simulink library "csc_peg_powered_explicit_guidance_lib"  (R2015b)
settings: Solver=VariableStepAuto  StartTime=0.0  StopTime=10.0  RelTol=1e-3
undefined symbols (not defined in the file or in its folder): accel, csc_gdn_dt, csc_peg_update_dt, DiscIntNeverNeededParam, gdn_landing_terminal_max_alt, gdn_millisec_per_cycle, gdn_peg_burn_cutoff_tgo, gdn_peg_pointing_hold_tgo, gdn_peg_Rmiss_tolerance, gdn_peg_thrust_gain, gdn_peg_Vmiss_tolerance, pos, tdl_main_biprop_thrust, tpl_main_biprop_isp, vel
libraries: util_common_lib x14, simulink x4, simulink_extras x3, util_info_lib x2, csu_arg_aimpoint_roll_guidance_lib x2, util_frame_rotation_lib x2, util_fsw_frame_rotation_lib x2, csc_peg_powered_explicit_guidance_lib x2, util_orbit_dynamics_lib x1, util_quat_lib x1
settings Model: Creator=Mark Agbayani  LastModifiedBy=Mark Agbayani

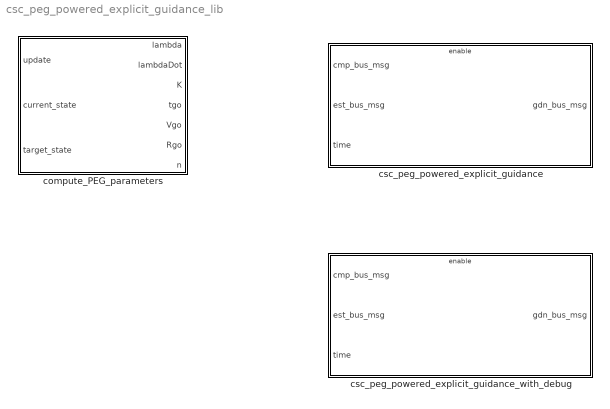
== system csc_peg_powered_explicit_guidance_lib ==
  compute_PEG_parameters : Subsystem  TreatAsAtomicUnit=on
  csc_peg_powered_explicit_guidance : Subsystem
  csc_peg_powered_explicit_guidance_with_debug : Subsystem

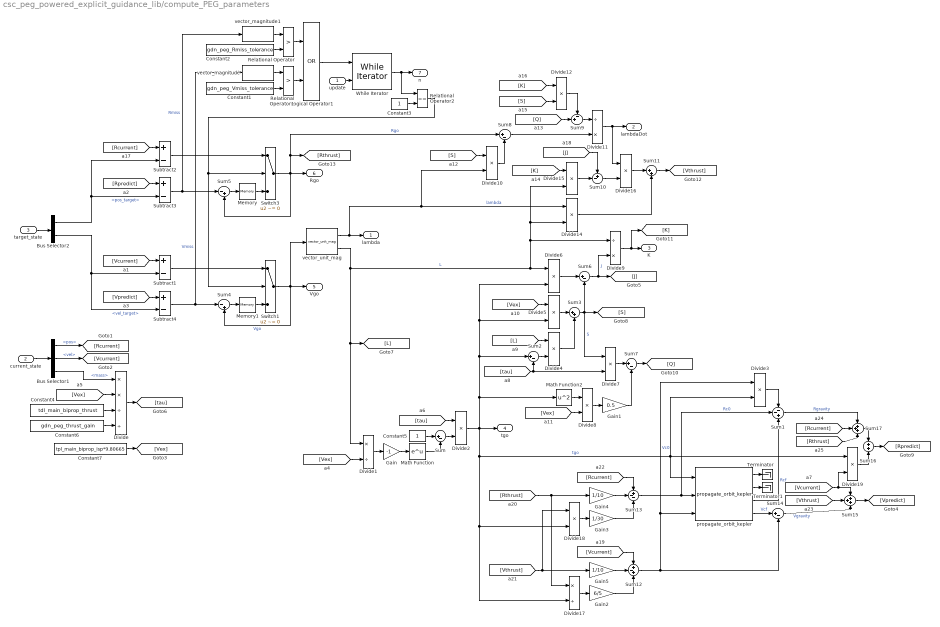
== system csc_peg_powered_explicit_guidance_lib/compute_PEG_parameters ==
  update : Inport
  current_state : Inport  Port=2
  target_state : Inport  Port=3
  Bus Selector1 : BusSelector  OutputSignals=pos,vel,mass
  Bus Selector2 : BusSelector  OutputSignals=pos_target,vel_target
  Constant1 : Constant  Value=gdn_peg_Vmiss_tolerance
  Constant2 : Constant  Value=gdn_peg_Rmiss_tolerance
  Constant3 : Constant
  Constant4 : Constant  Value=tdl_main_biprop_thrust
  Constant5 : Constant
  Constant6 : Constant  Value=gdn_peg_thrust_gain
  Constant7 : Constant  Value=tpl_main_biprop_isp*9.80665
  Divide : Product  Inputs=**//
  Divide1 : Product  Inputs=*/
  Divide{2..8,10,12,14..16,18..19} (14 alike) : Product  Inputs=**
  Divide11 : Product  Inputs=/*
  Divide17 : Product  Inputs=*/
  Divide9 : Product  Inputs=/*
  Gain : Gain  Gain=-1
  Gain1 : Gain  Gain=0.5
  Gain2 : Gain  Gain=6/5
  Gain3 : Gain  Gain=1/30
  Gain4 : Gain  Gain=1/10
  Gain5 : Gain  Gain=1/10
  Logical Operator1 : Logic  Operator=OR  AllPortsSameDT=off  OutDataTypeStr=boolean
  Math Function : Math  SaturateOnIntegerOverflow=on
  Math Function2 : Math  Operator=square  SaturateOnIntegerOverflow=on
  Memory : Memory  InheritSampleTime=on
  Memory1 : Memory  InheritSampleTime=on
  Relational Operator : RelationalOperator  Operator=>  OutDataTypeStr=boolean
  Relational Operator1 : RelationalOperator  Operator=>  OutDataTypeStr=boolean
  Relational Operator2 : RelationalOperator  Operator===  OutDataTypeStr=boolean
  Subtract{1..4} (4 alike) : Sum  Inputs=+-
  Sum{,2,6..8,14} (6 alike) : Sum  Inputs=|+-
  Sum1 : Sum  Inputs=--+
  Sum10 : Sum  Inputs=+-|
  Sum11 : Sum  Inputs=|++
  Sum12 : Sum  Inputs=+-+
  Sum13 : Sum  Inputs=+--
  Sum15 : Sum  Inputs=+++
  Sum16 : Sum  Inputs=+|+
  Sum17 : Sum  Inputs=+++
  Sum3 : Sum  Inputs=|++
  Sum4 : Sum  Inputs=|-+
  Sum5 : Sum  Inputs=|-+
  Sum9 : Sum  Inputs=-+|
  Switch1 : Switch  Criteria=u2 ~= 0
  Switch3 : Switch  Criteria=u2 ~= 0
  Terminator : Terminator
  Terminator1 : Terminator
  While Iterator : WhileIterator  MaxIters=gdn_peg_max_iterations  ResetStates=reset  ShowIterationPort=on  OutputDataType=double
  propagate_orbit_kepler : util_orbit_dynamics_lib/propagate_orbit_kepler
  vector_magnitude : util_common_lib/vector_magnitude  SystemSampleTime=-1
  vector_magnitude1 : util_common_lib/vector_magnitude  SystemSampleTime=-1
  vector_unit_mag : util_common_lib/vector_unit_mag  SystemSampleTime=-1
  lambda : Outport
  lambdaDot : Outport  Port=2
  K : Outport  Port=3
  tgo : Outport  Port=4
  Vgo : Outport  Port=5
  Rgo : Outport  Port=6
  n : Outport  Port=7
  wires:
  Constant6/1 -> Divide/4
  [Vex] -> Divide/2
  Constant4/1 -> Divide/3
  While Iterator/1 -> n/1, Relational Operator2/1
  propagate_orbit_kepler/2 -> Terminator1/1
  propagate_orbit_kepler/1 -> Terminator/1
  [Rthrust] -> Sum17/3
  [Rcurrent] -> Sum17/2
  Sum17/1 -> Sum16/1
  [Vthrust] -> Sum15/2
  Relational Operator1/1 -> Logical Operator1/2
  Relational Operator/1 -> Logical Operator1/1
  Sum15/1 -> [Vpredict]
  Sum16/1 -> [Rpredict]
  Divide19/1 -> Sum16/2
  Sum1/1 -> Sum17/1  "Rgravity"
  [Vcurrent] -> Sum15/1, Divide19/2
  Sum14/1 -> Sum15/3  "Vgravity"
  propagate_orbit_kepler/3 -> Sum1/3  "Rcf"
  Divide3/1 -> Sum1/1
  propagate_orbit_kepler/4 -> Sum14/1  "Vcf"
  Sum13/1 -> Sum1/2, propagate_orbit_kepler/2  "Rc0"
  Sum12/1 -> Sum14/2, Divide3/1, propagate_orbit_kepler/3  "Vc0"
  [Rcurrent] -> Sum13/1
  Gain3/1 -> Sum13/3
  Gain4/1 -> Sum13/2
  Gain5/1 -> Sum12/2
  Gain2/1 -> Sum12/3
  [Vcurrent] -> Sum12/1
  [Vthrust] -> Divide18/1, Gain5/1
  Divide18/1 -> Gain3/1
  [Rthrust] -> Divide17/1, Gain4/1
  Divide17/1 -> Gain2/1
  Sum11/1 -> [Vthrust]
  Divide9/1 -> K/1, [K]
  Divide15/1 -> Sum10/2
  [J] -> Sum10/1
  [K] -> Divide12/1
  [K] -> Divide15/1
  Divide14/1 -> Sum11/2
  Divide16/1 -> Sum11/1
  Sum6/1 -> [J], Divide9/2  "J"
  Sum10/1 -> Divide16/2
  Divide11/1 -> lambdaDot/1, Divide16/1
  vector_unit_mag/2 -> [L], Divide1/1, Divide6/1, Divide9/1, Divide14/2, Divide15/2  "L"
  [Q] -> Sum9/2
  Divide12/1 -> Sum9/1
  Sum9/1 -> Divide11/1
  [S] -> Divide12/2
  Sum8/1 -> Divide11/2
  Divide10/1 -> Sum8/2
  [S] -> Divide10/1
  Sum7/1 -> [Q]
  Gain1/1 -> Sum7/2
  Divide8/1 -> Gain1/1
  [Vex] -> Divide8/2
  Math Function2/1 -> Divide8/1
  Divide7/1 -> Sum7/1
  Divide6/1 -> Sum6/1
  Sum5/1 -> Memory/1
  Subtract3/1 -> Sum5/1, vector_magnitude1/1  "Rmiss"
  [Vpredict] -> Subtract4/1
  Subtract4/1 -> vector_magnitude/1, Sum4/1  "Vmiss"
  [Rpredict] -> Subtract3/1
  Sum3/1 -> Sum6/2, [S], Divide7/1  "S"
  Divide5/1 -> Sum3/1
  Divide4/1 -> Sum3/2
  [Vex] -> Divide5/1
  [L] -> Divide4/1
  Sum2/1 -> Divide4/2
  [tau] -> Divide7/2, Sum2/2
  Divide2/1 -> Math Function2/1, Sum2/1, Divide5/2, Divide6/2, propagate_orbit_kepler/1, Divide19/1, Divide3/2, Divide18/2, Divide17/2, tgo/1  "tgo"
  Math Function/1 -> Sum/2
  Constant5/1 -> Sum/1
  [tau] -> Divide2/1
  Divide1/1 -> Gain/1
  Gain/1 -> Math Function/1
  Constant7/1 -> [Vex]
  Sum/1 -> Divide2/2
  [Vex] -> Divide1/2
  Divide/1 -> [tau]
  Switch1/1 -> vector_unit_mag/1, Vgo/1, Sum4/2  "Vgo"
  Switch3/1 -> Sum5/2, Sum8/1, [Rthrust], Rgo/1  "Rgo"
  [Rcurrent] -> Subtract2/1
  [Vcurrent] -> Subtract1/1
  Bus Selector1/2 -> [Vcurrent]  "<vel>"
  Bus Selector1/1 -> [Rcurrent]  "<pos>"
  Bus Selector2/2 -> Subtract1/2, Subtract4/2  "<vel_target>"
  Bus Selector2/1 -> Subtract2/2, Subtract3/2  "<pos_target>"
  Subtract1/1 -> Switch1/1
  Subtract2/1 -> Switch3/1
  Relational Operator2/1 -> Switch1/2, Switch3/2
  Bus Selector1/3 -> Divide/1  "<mass>"
  target_state/1 -> Bus Selector2/1
  current_state/1 -> Bus Selector1/1
  Constant3/1 -> Relational Operator2/2
  vector_magnitude/1 -> Relational Operator1/1
  vector_magnitude1/1 -> Relational Operator/1
  Constant1/1 -> Relational Operator1/2
  Constant2/1 -> Relational Operator/2
  Logical Operator1/1 -> While Iterator/1
  update/1 -> While Iterator/2
  Memory/1 -> Switch3/3
  Sum4/1 -> Memory1/1
  Memory1/1 -> Switch1/3
  vector_unit_mag/1 -> lambda/1, Divide10/2, Divide14/1  "lambda"

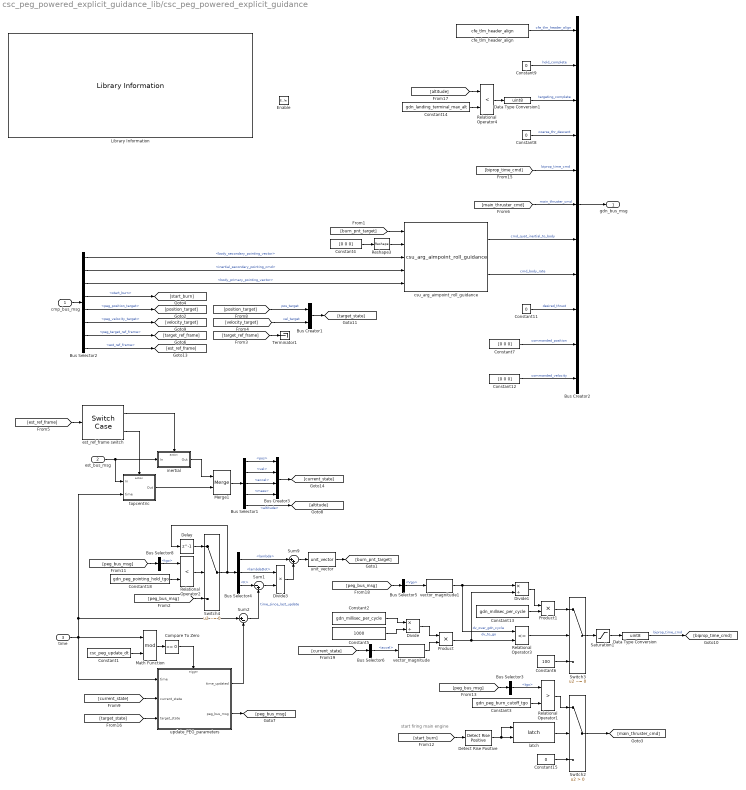
== system csc_peg_powered_explicit_guidance_lib/csc_peg_powered_explicit_guidance ==
  note: start firing main engine
  cmp_bus_msg : Inport
  est_bus_msg : Inport  Port=2
  time : Inport  Port=3
  Enable : EnablePort  StatesWhenEnabling=reset
  Bus Creator1 : BusCreator  Inputs=2
  Bus Creator3 : BusCreator  Inputs=4
  Bus Selector1 : BusSelector  OutputSignals=pos,vel,accel,mass,altitude
  Bus Selector2 : BusSelector  OutputSignals=body_secondary_pointing_vector,inertial_secondary_pointing_cmd,body_primary_pointing_vector,start_burn,peg_position_target,peg_velocity_target,peg_target_ref_frame,est_ref_frame
  Bus Selector3 : BusSelector  OutputSignals=tgo
  Bus Selector4 : BusSelector  OutputSignals=lambda,lambdaDot,K
  Bus Selector5 : BusSelector  OutputSignals=Vgo
  Bus Selector6 : BusSelector  OutputSignals=accel
  Bus Selector8 : BusSelector  OutputSignals=tgo
  Bus Creator2 : BusCreator  Inputs=11  OutDataTypeStr=Bus: gdn_bus_msg  NonVirtualBus=on
  Compare To Zero : simulink/Logic and Bit Operations/Compare To Zero  relop===  OutDataTypeStr=boolean
  Constant1 : Constant  Value=csc_peg_update_dt
  Constant11 : Constant  Value=0
  Constant12 : Constant  Value=[0 0 0]
  Constant13 : Constant  Value=gdn_millisec_per_cycle
  Constant14 : Constant  Value=gdn_landing_terminal_max_alt
  Constant15 : Constant  Value=0  OutDataTypeStr=double
  Constant18 : Constant  Value=gdn_peg_pointing_hold_tgo
  Constant2 : Constant  Value=gdn_millisec_per_cycle
  Constant3 : Constant  Value=gdn_peg_burn_cutoff_tgo
  Constant4 : Constant  Value=[0 0 0]
  Constant5 : Constant  Value=1000
  Constant6 : Constant  Value=100
  Constant7 : Constant  Value=[0 0 0]
  Constant8 : Constant  Value=0  OutDataTypeStr=uint8
  Constant9 : Constant  Value=0  OutDataTypeStr=uint8
  Data Type Conversion : DataTypeConversion  OutDataTypeStr=uint8
  Data Type Conversion1 : DataTypeConversion  OutDataTypeStr=uint8
  Delay : Delay  DelayLength=1  InitialCondition=0
  Detect Rise Positive : simulink/Logic and Bit Operations/Detect Rise Positive  vinit=0  InputProcessing=Inherited  OutDataTypeStr=boolean
  Divide : Product  Inputs=*/
  Divide1 : Product  Inputs=*/
  Divide3 : Product  Inputs=**  OutDataTypeStr=double
  Library Information : util_info_lib/Library Information  owner='jkaidy'
  Math Function : Math  Operator=mod  SaturateOnIntegerOverflow=on
  Merge1 : Merge  InitialOutput=0
  Product : Product
  Product1 : Product
  Relational Operator1 : RelationalOperator  Operator=>  OutDataTypeStr=boolean
  Relational Operator2 : RelationalOperator  Operator=<  OutDataTypeStr=boolean
  Relational Operator3 : RelationalOperator  Operator=<=  OutDataTypeStr=boolean
  Relational Operator4 : RelationalOperator  Operator=<  OutDataTypeStr=boolean
  Reshape3 : Reshape  OutputDimensionality=Column vector (2-D)
  Saturation1 : Saturate  UpperLimit=100  LowerLimit=0
  Sum1 : Sum  Inputs=|-+  AccumDataTypeStr=double
  Sum2 : Sum  Inputs=|+-
  Sum9 : Sum  Inputs=|++  AccumDataTypeStr=double
  Switch2 : Switch  Criteria=u2 > Threshold
  Switch3 : Switch  Criteria=u2 ~= 0
  Switch4 : Switch  Criteria=u2 ~= 0  OutDataTypeStr=double
  Terminator1 : Terminator
  cfe_tlm_header_align : util_common_lib/cfe_tlm_header_align
  csu_arg_aimpoint_roll_guidance : csu_arg_aimpoint_roll_guidance_lib/csu_arg_aimpoint_roll_guidance
  est_ref_frame switch : SwitchCase  CaseConditions={uint8(enum_reference_frame.inertial),uint8(enum_reference_frame.topocentric)}  ShowDefaultCase=off
  inertial : Subsystem  TreatAsAtomicUnit=on
  latch : util_common_lib/latch  Initial_Latch=0
  topcentric : Subsystem  TreatAsAtomicUnit=on
  unit_vector : util_common_lib/unit_vector  SystemSampleTime=-1
  update_PEG_parameters : Subsystem  TreatAsAtomicUnit=on
  vector_magnitude : util_common_lib/vector_magnitude  SystemSampleTime=-1
  vector_magnitude1 : util_common_lib/vector_magnitude  SystemSampleTime=-1
  gdn_bus_msg : Outport  OutDataTypeStr=Bus: gdn_bus_msg
  wires:
  Merge1/1 -> Bus Selector1/1
  [est_ref_frame] -> est_ref_frame switch/1
  time/1 -> update_PEG_parameters/1(time), Math Function/1, Sum2/1, topcentric/2(time)
  est_ref_frame switch/2 -> topcentric/Action
  topcentric/1(Out) -> Merge1/2
  inertial/1(Out) -> Merge1/1
  est_bus_msg/1 -> inertial/1(In), topcentric/1(In)
  est_ref_frame switch/1 -> inertial/Action
  [current_state] -> Bus Selector6/1
  Bus Creator3/1 -> [current_state]
  Bus Selector1/1 -> Bus Creator3/1  "<pos>"
  Bus Selector1/2 -> Bus Creator3/2  "<vel>"
  Bus Selector1/3 -> Bus Creator3/3  "<accel>"
  Bus Selector2/8 -> [est_ref_frame]  "<est_ref_frame>"
  Bus Selector2/7 -> [target_ref_frame]  "<peg_target_ref_frame>"
  Bus Creator1/1 -> [target_state]
  [position_target] -> Bus Creator1/1  "pos_target"
  [velocity_target] -> Bus Creator1/2  "vel_target"
  [target_ref_frame] -> Terminator1/1
  [biprop_time_cmd] -> Bus Creator2/5  "biprop_time_cmd"
  cmp_bus_msg/1 -> Bus Selector2/1
  Bus Selector2/5 -> [position_target]  "<peg_position_target>"
  Bus Selector2/6 -> [velocity_target]  "<peg_velocity_target>"
  Bus Selector2/1 -> csu_arg_aimpoint_roll_guidance/3  "<body_secondary_pointing_vector>"
  Bus Selector2/2 -> csu_arg_aimpoint_roll_guidance/4  "<inertial_secondary_pointing_cmd>"
  Bus Selector2/3 -> csu_arg_aimpoint_roll_guidance/5  "<body_primary_pointing_vector>"
  Bus Selector2/4 -> [start_burn]  "<start_burn>"
  Constant11/1 -> Bus Creator2/9  "desired_thrust"
  Constant8/1 -> Bus Creator2/4  "coarse_thr_descent"
  [main_thruster_cmd] -> Bus Creator2/6  "main_thruster_cmd"
  csu_arg_aimpoint_roll_guidance/1 -> Bus Creator2/7  "cmd_quat_inertial_to_body"
  csu_arg_aimpoint_roll_guidance/2 -> Bus Creator2/8  "cmd_body_rate"
  Constant9/1 -> Bus Creator2/2  "hold_complete"
  Data Type Conversion1/1 -> Bus Creator2/3  "targeting_complete"
  cfe_tlm_header_align/1 -> Bus Creator2/1  "cfe_tlm_header_align"
  Constant12/1 -> Bus Creator2/11  "commanded_velocity"
  Constant7/1 -> Bus Creator2/10  "commanded_position"
  Detect Rise Positive/1 -> latch/1, latch/2
  [start_burn] -> Detect Rise Positive/1
  Constant3/1 -> Relational Operator1/2
  Relational Operator1/1 -> Switch2/1
  Constant15/1 -> Switch2/3
  Switch2/1 -> [main_thruster_cmd]
  latch/1 -> Switch2/2
  Bus Selector1/4 -> Bus Creator3/4  "<mass>"
  [burn_pnt_target] -> csu_arg_aimpoint_roll_guidance/1
  Reshape3/1 -> csu_arg_aimpoint_roll_guidance/2
  Constant4/1 -> Reshape3/1
  [current_state] -> update_PEG_parameters/2(current_state)
  [target_state] -> update_PEG_parameters/3(target_state)
  Bus Selector3/1 -> Relational Operator1/1  "<tgo>"
  [peg_bus_msg] -> Bus Selector3/1
  update_PEG_parameters/2(peg_bus_msg) -> [peg_bus_msg]
  Math Function/1 -> Compare To Zero/1
  Constant1/1 -> Math Function/2
  update_PEG_parameters/1(time_updated) -> Sum2/2
  Data Type Conversion/1 -> [biprop_time_cmd]  "biprop_time_cmd"
  Saturation1/1 -> Data Type Conversion/1
  vector_magnitude/1 -> Product/2
  Switch3/1 -> Saturation1/1
  Product1/1 -> Switch3/1
  Divide1/1 -> Product1/1
  Constant13/1 -> Product1/2
  Product/1 -> Relational Operator3/2, Divide1/2  "dv_over_gdn_cycle"
  Constant6/1 -> Switch3/3
  Relational Operator3/1 -> Switch3/2
  vector_magnitude1/1 -> Relational Operator3/1, Divide1/1  "dv_to_go"
  Bus Selector6/1 -> vector_magnitude/1  "<accel>"
  Divide/1 -> Product/1
  Constant5/1 -> Divide/2
  Constant2/1 -> Divide/1
  [peg_bus_msg] -> Bus Selector5/1
  Bus Selector5/1 -> vector_magnitude1/1  "<Vgo>"
  Bus Creator2/1 -> gdn_bus_msg/1
  Compare To Zero/1 -> update_PEG_parameters/Trigger
  unit_vector/1 -> [burn_pnt_target]
  Bus Selector1/5 -> [altitude]  "<altitude>"
  [altitude] -> Relational Operator4/1
  Constant14/1 -> Relational Operator4/2
  Relational Operator4/1 -> Data Type Conversion1/1
  Sum2/1 -> Sum1/2  "time_since_last_update"
  Switch4/1 -> Delay/1, Bus Selector4/1
  Sum1/1 -> Divide3/2
  Divide3/1 -> Sum9/2
  Bus Selector4/3 -> Sum1/1  "<K>"
  Bus Selector4/2 -> Divide3/1  "<lambdaDot>"
  Bus Selector4/1 -> Sum9/1  "<lambda>"
  Sum9/1 -> unit_vector/1
  Bus Selector8/1 -> Relational Operator2/1  "<tgo>"
  [peg_bus_msg] -> Bus Selector8/1
  Constant18/1 -> Relational Operator2/2
  Delay/1 -> Switch4/1
  Relational Operator2/1 -> Switch4/2
  [peg_bus_msg] -> Switch4/3

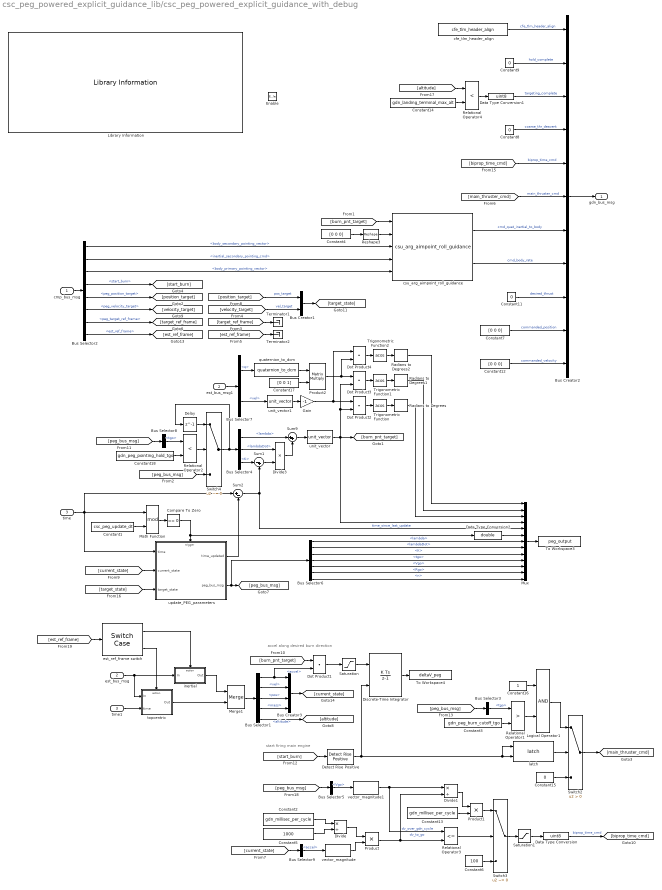
== system csc_peg_powered_explicit_guidance_lib/csc_peg_powered_explicit_guidance_with_debug ==
  note: accel along desired burn direction
  note: start firing main engine
  cmp_bus_msg : Inport
  est_bus_msg : Inport  Port=2
  time : Inport  Port=3
  Enable : EnablePort  StatesWhenEnabling=reset
  Bus Creator1 : BusCreator  Inputs=2
  Bus Creator3 : BusCreator  Inputs=4
  Bus Selector1 : BusSelector  OutputSignals=accel,vel,pos,mass,altitude
  Bus Selector2 : BusSelector  OutputSignals=body_secondary_pointing_vector,inertial_secondary_pointing_cmd,body_primary_pointing_vector,start_burn,peg_position_target,peg_velocity_target,peg_target_ref_frame,est_ref_frame
  Bus Selector3 : BusSelector  OutputSignals=tgo
  Bus Selector4 : BusSelector  OutputSignals=lambda,lambdaDot,K
  Bus Selector5 : BusSelector  OutputSignals=Vgo
  Bus Selector6 : BusSelector  OutputSignals=lambda,lambdaDot,K,tgo,Vgo,Rgo,n
  Bus Selector7 : BusSelector  OutputSignals=q,vel
  Bus Selector8 : BusSelector  OutputSignals=tgo
  Bus Selector9 : BusSelector  OutputSignals=accel
  Bus Creator2 : BusCreator  Inputs=11  OutDataTypeStr=Bus: gdn_bus_msg  NonVirtualBus=on
  Compare To Zero : simulink/Logic and Bit Operations/Compare To Zero  relop===  OutDataTypeStr=boolean
  Constant1 : Constant  Value=csc_peg_update_dt
  Constant11 : Constant  Value=0
  Constant12 : Constant  Value=[0 0 0]
  Constant13 : Constant  Value=gdn_millisec_per_cycle
  Constant14 : Constant  Value=gdn_landing_terminal_max_alt
  Constant15 : Constant  Value=0  OutDataTypeStr=double
  Constant16 : Constant  OutDataTypeStr=boolean
  Constant17 : Constant  Value=[0 0 1]
  Constant18 : Constant  Value=gdn_peg_pointing_hold_tgo
  Constant2 : Constant  Value=gdn_millisec_per_cycle
  Constant3 : Constant  Value=gdn_peg_burn_cutoff_tgo
  Constant4 : Constant  Value=[0 0 0]
  Constant5 : Constant  Value=1000
  Constant6 : Constant  Value=100
  Constant7 : Constant  Value=[0 0 0]
  Constant8 : Constant  Value=0  OutDataTypeStr=uint8
  Constant9 : Constant  Value=0  OutDataTypeStr=uint8
  Data Type Conversion : DataTypeConversion  OutDataTypeStr=uint8
  Data Type Conversion1 : DataTypeConversion  OutDataTypeStr=uint8
  Data Type Conversion2 : DataTypeConversion  OutDataTypeStr=double
  Delay : Delay  DelayLength=1  InitialCondition=0
  Detect Rise Positive : simulink/Logic and Bit Operations/Detect Rise Positive  vinit=0  InputProcessing=Inherited  OutDataTypeStr=boolean
  Discrete-Time Integrator : DiscreteIntegrator  ExternalReset=rising  SampleTime=csc_gdn_dt  ICPrevOutput=DiscIntNeverNeededParam  ICPrevScaledInput=DiscIntNeverNeededParam
  Divide : Product  Inputs=*/
  Divide1 : Product  Inputs=*/
  Divide3 : Product  Inputs=**  OutDataTypeStr=double
  Dot Product{1..4} (4 alike) : DotProduct  InputSameDT=on  OutDataTypeStr=Inherit: Inherit via internal rule
  Gain : Gain  Gain=-1
  Library Information : util_info_lib/Library Information  owner='jkaidy'
  Logical Operator1 : Logic  AllPortsSameDT=off  OutDataTypeStr=boolean
  Math Function : Math  Operator=mod  SaturateOnIntegerOverflow=on
  Merge1 : Merge  InitialOutput=0
  Mux : Mux  Inputs=13
  Product : Product
  Product1 : Product
  Product2 : Product  Multiplication=Matrix(*)  RndMeth=Zero
  Radians to Degrees : simulink_extras/Transformations/Radians to Degrees
  Radians to Degrees1 : simulink_extras/Transformations/Radians to Degrees
  Radians to Degrees2 : simulink_extras/Transformations/Radians to Degrees
  Relational Operator1 : RelationalOperator  Operator=>  OutDataTypeStr=boolean
  Relational Operator2 : RelationalOperator  Operator=<  OutDataTypeStr=boolean
  Relational Operator3 : RelationalOperator  Operator=<=  OutDataTypeStr=boolean
  Relational Operator4 : RelationalOperator  Operator=<  OutDataTypeStr=boolean
  Reshape3 : Reshape  OutputDimensionality=Column vector (2-D)
  Saturation : Saturate  UpperLimit=1e6  LowerLimit=0
  Saturation1 : Saturate  UpperLimit=100  LowerLimit=0
  Sum1 : Sum  Inputs=|-+  AccumDataTypeStr=double
  Sum2 : Sum  Inputs=|+-
  Sum9 : Sum  Inputs=|++  AccumDataTypeStr=double
  Switch2 : Switch  Criteria=u2 > Threshold
  Switch3 : Switch  Criteria=u2 ~= 0
  Switch4 : Switch  Criteria=u2 ~= 0  OutDataTypeStr=double
  Terminator1 : Terminator
  Terminator2 : Terminator
  To Workspace3 : ToWorkspace  VariableName=peg_output  SaveFormat=Structure With Time  SampleTime=-1
  To Workspace4 : ToWorkspace  VariableName=deltaV_peg  SaveFormat=Structure With Time  SampleTime=-1
  Trigonometric Function : Trigonometry  Operator=acos
  Trigonometric Function1 : Trigonometry  Operator=acos
  Trigonometric Function2 : Trigonometry  Operator=acos
  cfe_tlm_header_align : util_common_lib/cfe_tlm_header_align
  csu_arg_aimpoint_roll_guidance : csu_arg_aimpoint_roll_guidance_lib/csu_arg_aimpoint_roll_guidance
  est_bus_msg1 : InportShadow  Port=2
  est_ref_frame switch : SwitchCase  CaseConditions={uint8(enum_reference_frame.inertial),uint8(enum_reference_frame.topocentric)}  ShowDefaultCase=off
  inertial : Subsystem  TreatAsAtomicUnit=on
  latch : util_common_lib/latch  Initial_Latch=0
  quaternion_to_dcm : util_quat_lib/quaternion_to_dcm  SystemSampleTime=-1
  time1 : InportShadow  Port=3
  topcentric : Subsystem  TreatAsAtomicUnit=on
  unit_vector : util_common_lib/unit_vector  SystemSampleTime=-1
  unit_vector1 : util_common_lib/unit_vector  SystemSampleTime=-1
  update_PEG_parameters : Subsystem  TreatAsAtomicUnit=on
  vector_magnitude : util_common_lib/vector_magnitude  SystemSampleTime=-1
  vector_magnitude1 : util_common_lib/vector_magnitude  SystemSampleTime=-1
  gdn_bus_msg : Outport  OutDataTypeStr=Bus: gdn_bus_msg
  wires:
  [current_state] -> Bus Selector9/1
  time1/1 -> topcentric/2(time)
  Bus Selector1/1 -> Bus Creator3/1, Dot Product1/2  "<accel>"
  Bus Selector1/2 -> Bus Creator3/2  "<vel>"
  Bus Selector1/3 -> Bus Creator3/3  "<pos>"
  [est_ref_frame] -> Terminator2/1
  Bus Selector2/8 -> [est_ref_frame]  "<est_ref_frame>"
  Constant16/1 -> Logical Operator1/1
  Relational Operator1/1 -> Logical Operator1/2
  [peg_bus_msg] -> Bus Selector3/1
  Bus Selector3/1 -> Relational Operator1/1  "<tgo>"
  Constant3/1 -> Relational Operator1/2
  Dot Product4/1 -> Trigonometric Function2/1
  Trigonometric Function2/1 -> Radians to Degrees2/1
  Saturation/1 -> Discrete-Time Integrator/1
  [burn_pnt_target] -> Dot Product1/1
  Dot Product1/1 -> Saturation/1
  Detect Rise Positive/1 -> latch/2, latch/1, Discrete-Time Integrator/2
  Discrete-Time Integrator/1 -> To Workspace4/1
  update_PEG_parameters/2(peg_bus_msg) -> [peg_bus_msg], Bus Selector6/1
  Sum2/1 -> Sum1/2, Mux/5  "time_since_last_update"
  Mux/1 -> To Workspace3/1
  unit_vector/1 -> Dot Product3/2, Dot Product2/2, [burn_pnt_target], Mux/4
  Bus Selector6/1 -> Mux/7  "<lambda>"
  Bus Selector6/2 -> Mux/8  "<lambdaDot>"
  Bus Selector6/3 -> Mux/9  "<K>"
  Bus Selector6/4 -> Mux/10  "<tgo>"
  Bus Selector6/5 -> Mux/11  "<Vgo>"
  Bus Selector6/6 -> Mux/12  "<Rgo>"
  Bus Selector6/7 -> Mux/13  "<n>"
  Compare To Zero/1 -> update_PEG_parameters/Trigger, Data Type Conversion2/1
  Data Type Conversion2/1 -> Mux/6
  est_bus_msg1/1 -> Bus Selector7/1
  Bus Selector7/2 -> unit_vector1/1  "<vel>"
  unit_vector1/1 -> Gain/1
  Dot Product2/1 -> Trigonometric Function/1
  Trigonometric Function/1 -> Radians to Degrees/1
  Radians to Degrees/1 -> Mux/3
  Gain/1 -> Dot Product2/1, Dot Product4/1
  Bus Selector7/1 -> quaternion_to_dcm/1  "<q>"
  quaternion_to_dcm/1 -> Product2/1
  Constant17/1 -> Product2/2
  Dot Product3/1 -> Trigonometric Function1/1
  Trigonometric Function1/1 -> Radians to Degrees1/1
  Radians to Degrees1/1 -> Mux/2
  Product2/1 -> Dot Product4/2, Dot Product3/1
  Radians to Degrees2/1 -> Mux/1
  [target_ref_frame] -> Terminator1/1
  Bus Selector2/6 -> [velocity_target]  "<peg_velocity_target>"
  Bus Selector2/7 -> [target_ref_frame]  "<peg_target_ref_frame>"
  Bus Selector2/5 -> [position_target]  "<peg_position_target>"
  Bus Creator2/1 -> gdn_bus_msg/1
  Bus Selector5/1 -> vector_magnitude1/1  "<Vgo>"
  [peg_bus_msg] -> Bus Selector5/1
  Constant2/1 -> Divide/1
  Constant5/1 -> Divide/2
  Divide/1 -> Product/1
  Bus Selector9/1 -> vector_magnitude/1  "<accel>"
  Product/1 -> Relational Operator3/2, Divide1/2  "dv_over_gdn_cycle"
  vector_magnitude1/1 -> Divide1/1, Relational Operator3/1  "dv_to_go"
  Relational Operator3/1 -> Switch3/2
  Constant6/1 -> Switch3/3
  Constant13/1 -> Product1/2
  Divide1/1 -> Product1/1
  Product1/1 -> Switch3/1
  Switch3/1 -> Saturation1/1
  vector_magnitude/1 -> Product/2
  Saturation1/1 -> Data Type Conversion/1
  Data Type Conversion/1 -> [biprop_time_cmd]  "biprop_time_cmd"
  update_PEG_parameters/1(time_updated) -> Sum2/2
  time/1 -> Sum2/1, Math Function/1, update_PEG_parameters/1(time)
  Constant1/1 -> Math Function/2
  Math Function/1 -> Compare To Zero/1
  [velocity_target] -> Bus Creator1/2  "vel_target"
  [position_target] -> Bus Creator1/1  "pos_target"
  Bus Creator1/1 -> [target_state]
  [target_state] -> update_PEG_parameters/3(target_state)
  [current_state] -> update_PEG_parameters/2(current_state)
  Constant4/1 -> Reshape3/1
  Reshape3/1 -> csu_arg_aimpoint_roll_guidance/2
  [burn_pnt_target] -> csu_arg_aimpoint_roll_guidance/1
  latch/1 -> Switch2/2
  Switch2/1 -> [main_thruster_cmd]
  Constant15/1 -> Switch2/3
  Logical Operator1/1 -> Switch2/1
  [start_burn] -> Detect Rise Positive/1
  Constant7/1 -> Bus Creator2/10  "commanded_position"
  Constant12/1 -> Bus Creator2/11  "commanded_velocity"
  cfe_tlm_header_align/1 -> Bus Creator2/1  "cfe_tlm_header_align"
  Data Type Conversion1/1 -> Bus Creator2/3  "targeting_complete"
  csu_arg_aimpoint_roll_guidance/2 -> Bus Creator2/8  "cmd_body_rate"
  csu_arg_aimpoint_roll_guidance/1 -> Bus Creator2/7  "cmd_quat_inertial_to_body"
  [main_thruster_cmd] -> Bus Creator2/6  "main_thruster_cmd"
  Constant8/1 -> Bus Creator2/4  "coarse_thr_descent"
  Constant11/1 -> Bus Creator2/9  "desired_thrust"
  Bus Selector2/4 -> [start_burn]  "<start_burn>"
  Bus Selector2/3 -> csu_arg_aimpoint_roll_guidance/5  "<body_primary_pointing_vector>"
  Bus Selector2/2 -> csu_arg_aimpoint_roll_guidance/4  "<inertial_secondary_pointing_cmd>"
  Bus Selector2/1 -> csu_arg_aimpoint_roll_guidance/3  "<body_secondary_pointing_vector>"
  cmp_bus_msg/1 -> Bus Selector2/1
  [biprop_time_cmd] -> Bus Creator2/5  "biprop_time_cmd"
  [altitude] -> Relational Operator4/1
  Constant14/1 -> Relational Operator4/2
  Relational Operator4/1 -> Data Type Conversion1/1
  Constant9/1 -> Bus Creator2/2  "hold_complete"
  Switch4/1 -> Delay/1, Bus Selector4/1
  Sum1/1 -> Divide3/2
  Divide3/1 -> Sum9/2
  Bus Selector4/3 -> Sum1/1  "<K>"
  Bus Selector4/2 -> Divide3/1  "<lambdaDot>"
  Bus Selector4/1 -> Sum9/1  "<lambda>"
  Sum9/1 -> unit_vector/1
  Bus Selector8/1 -> Relational Operator2/1  "<tgo>"
  [peg_bus_msg] -> Bus Selector8/1
  Constant18/1 -> Relational Operator2/2
  Delay/1 -> Switch4/1
  Relational Operator2/1 -> Switch4/2
  [peg_bus_msg] -> Switch4/3
  Bus Selector1/5 -> [altitude]  "<altitude>"
  Bus Selector1/4 -> Bus Creator3/4  "<mass>"
  Bus Creator3/1 -> [current_state]
  est_ref_frame switch/1 -> inertial/Action
  est_bus_msg/1 -> topcentric/1(In), inertial/1(In)
  inertial/1(Out) -> Merge1/1
  topcentric/1(Out) -> Merge1/2
  est_ref_frame switch/2 -> topcentric/Action
  [est_ref_frame] -> est_ref_frame switch/1
  Merge1/1 -> Bus Selector1/1

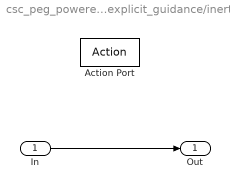
== system csc_peg_powered_explicit_guidance_lib/csc_peg_powered_explicit_guidance/inertial ==
  In : Inport
  Action Port : ActionPort
  Out : Outport
  wires:
  In/1 -> Out/1

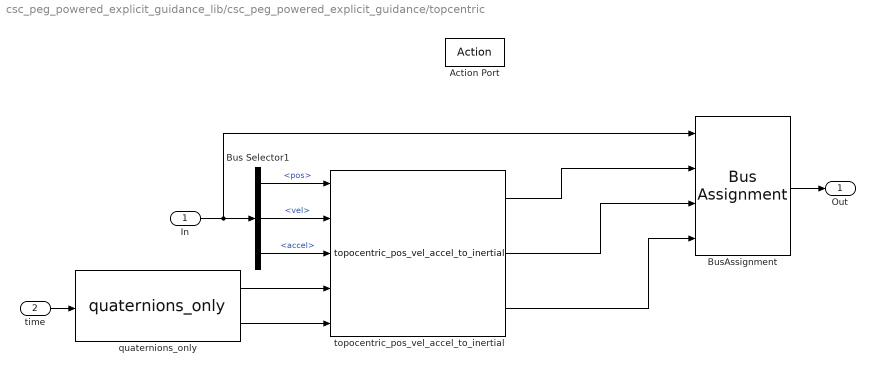
== system csc_peg_powered_explicit_guidance_lib/csc_peg_powered_explicit_guidance/topcentric ==
  In : Inport
  time : Inport  Port=2
  Action Port : ActionPort
  Bus Selector1 : BusSelector  OutputSignals=pos,vel,accel
  BusAssignment : BusAssignment  AssignedSignals=pos,vel,accel
  quaternions_only : util_frame_rotation_lib/quaternions_only  SystemSampleTime=-1
  topocentric_pos_vel_accel_to_inertial : util_fsw_frame_rotation_lib/topocentric_pos_vel_accel_to_inertial  SystemSampleTime=-1
  Out : Outport
  wires:
  quaternions_only/2 -> topocentric_pos_vel_accel_to_inertial/5
  quaternions_only/1 -> topocentric_pos_vel_accel_to_inertial/4
  time/1 -> quaternions_only/1
  BusAssignment/1 -> Out/1
  topocentric_pos_vel_accel_to_inertial/3 -> BusAssignment/4
  topocentric_pos_vel_accel_to_inertial/2 -> BusAssignment/3
  topocentric_pos_vel_accel_to_inertial/1 -> BusAssignment/2
  In/1 -> Bus Selector1/1, BusAssignment/1
  Bus Selector1/3 -> topocentric_pos_vel_accel_to_inertial/3  "<accel>"
  Bus Selector1/2 -> topocentric_pos_vel_accel_to_inertial/2  "<vel>"
  Bus Selector1/1 -> topocentric_pos_vel_accel_to_inertial/1  "<pos>"

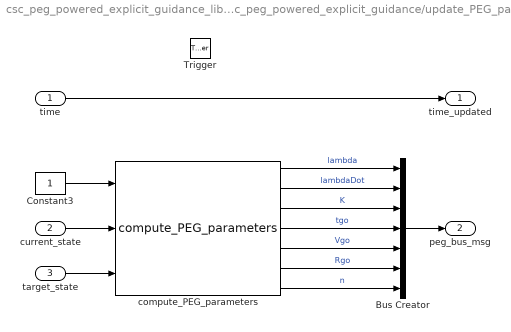
== system csc_peg_powered_explicit_guidance_lib/csc_peg_powered_explicit_guidance/update_PEG_parameters ==
  time : Inport
  current_state : Inport  Port=2
  target_state : Inport  Port=3
  Trigger : TriggerPort  TriggerType=falling
  Bus Creator : BusCreator  Inputs=7
  Constant3 : Constant
  compute_PEG_parameters : csc_peg_powered_explicit_guidance_lib/compute_PEG_parameters
  time_updated : Outport
  peg_bus_msg : Outport  Port=2
  wires:
  compute_PEG_parameters/4 -> Bus Creator/4  "tgo"
  compute_PEG_parameters/7 -> Bus Creator/7  "n"
  compute_PEG_parameters/6 -> Bus Creator/6  "Rgo"
  compute_PEG_parameters/5 -> Bus Creator/5  "Vgo"
  compute_PEG_parameters/3 -> Bus Creator/3  "K"
  compute_PEG_parameters/2 -> Bus Creator/2  "lambdaDot"
  compute_PEG_parameters/1 -> Bus Creator/1  "lambda"
  Bus Creator/1 -> peg_bus_msg/1
  current_state/1 -> compute_PEG_parameters/2
  target_state/1 -> compute_PEG_parameters/3
  Constant3/1 -> compute_PEG_parameters/1
  time/1 -> time_updated/1

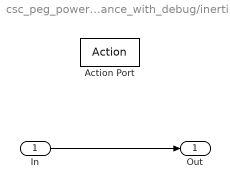
== system csc_peg_powered_explicit_guidance_lib/csc_peg_powered_explicit_guidance_with_debug/inertial ==
  In : Inport
  Action Port : ActionPort
  Out : Outport
  wires:
  In/1 -> Out/1

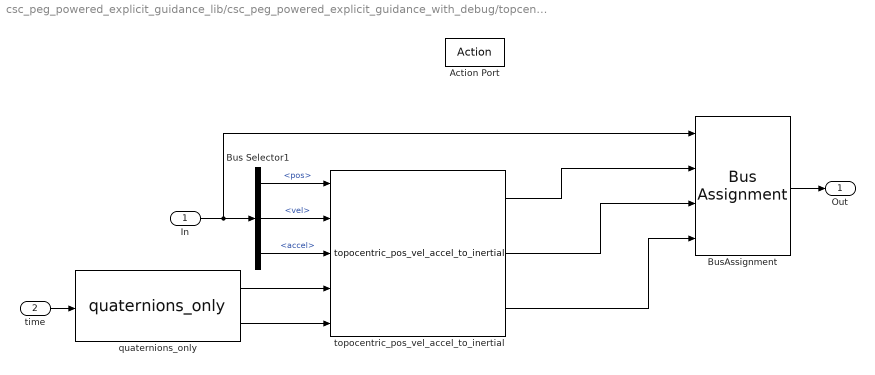
== system csc_peg_powered_explicit_guidance_lib/csc_peg_powered_explicit_guidance_with_debug/topcentric ==
  In : Inport
  time : Inport  Port=2
  Action Port : ActionPort
  Bus Selector1 : BusSelector  OutputSignals=pos,vel,accel
  BusAssignment : BusAssignment  AssignedSignals=pos,vel,accel
  quaternions_only : util_frame_rotation_lib/quaternions_only  SystemSampleTime=-1
  topocentric_pos_vel_accel_to_inertial : util_fsw_frame_rotation_lib/topocentric_pos_vel_accel_to_inertial  SystemSampleTime=-1
  Out : Outport
  wires:
  Bus Selector1/1 -> topocentric_pos_vel_accel_to_inertial/1  "<pos>"
  Bus Selector1/2 -> topocentric_pos_vel_accel_to_inertial/2  "<vel>"
  Bus Selector1/3 -> topocentric_pos_vel_accel_to_inertial/3  "<accel>"
  In/1 -> BusAssignment/1, Bus Selector1/1
  topocentric_pos_vel_accel_to_inertial/1 -> BusAssignment/2
  topocentric_pos_vel_accel_to_inertial/2 -> BusAssignment/3
  topocentric_pos_vel_accel_to_inertial/3 -> BusAssignment/4
  BusAssignment/1 -> Out/1
  time/1 -> quaternions_only/1
  quaternions_only/1 -> topocentric_pos_vel_accel_to_inertial/4
  quaternions_only/2 -> topocentric_pos_vel_accel_to_inertial/5

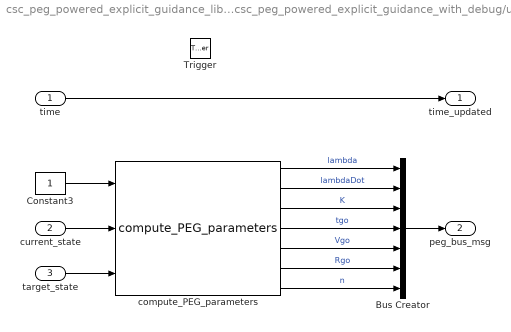
== system csc_peg_powered_explicit_guidance_lib/csc_peg_powered_explicit_guidance_with_debug/update_PEG_parameters ==
  time : Inport
  current_state : Inport  Port=2
  target_state : Inport  Port=3
  Trigger : TriggerPort  TriggerType=falling
  Bus Creator : BusCreator  Inputs=7
  Constant3 : Constant
  compute_PEG_parameters : csc_peg_powered_explicit_guidance_lib/compute_PEG_parameters
  time_updated : Outport
  peg_bus_msg : Outport  Port=2
  wires:
  time/1 -> time_updated/1
  Constant3/1 -> compute_PEG_parameters/1
  target_state/1 -> compute_PEG_parameters/3
  current_state/1 -> compute_PEG_parameters/2
  Bus Creator/1 -> peg_bus_msg/1
  compute_PEG_parameters/1 -> Bus Creator/1  "lambda"
  compute_PEG_parameters/2 -> Bus Creator/2  "lambdaDot"
  compute_PEG_parameters/3 -> Bus Creator/3  "K"
  compute_PEG_parameters/5 -> Bus Creator/5  "Vgo"
  compute_PEG_parameters/6 -> Bus Creator/6  "Rgo"
  compute_PEG_parameters/7 -> Bus Creator/7  "n"
  compute_PEG_parameters/4 -> Bus Creator/4  "tgo"
